simulink model "full_obs_res_gen_sim"  (R2020a)
settings: Solver=VariableStepAuto  StartTime=0.0  StopTime=15.0  RelTol=1e-3
values from neighbouring files (symbols this model uses):
  A = [ [0.5,1,0]; [1, 0, -1]; [1, 1, -0.5] ]    [init_demo_plant.m]    (also in init_demo_plant_2.m = [ [0.5,0.41,0.7]; [0.75, 0, -1.8]; [1.1, 0.8, -0.5] ])
  B = [ [1, -1]; [0, 1]; [1, 0] ]    [init_demo_plant.m]    (also in init_demo_plant_2.m = [ [0.1, -0.2, 0.3]; [0.5, 0.1, 0.35]; [1, 0, 0.7] ])
  C = [ [1, 0, 0]; [0, 0, 1] ]    [init_demo_plant.m]    (also in init_demo_plant_2.m = [ [1, 0, 0]; [0, 0, 1]; [0, 1, 0] ])
  D = [ [0, 0]; [0, 0] ]    [init_demo_plant.m]    (also in init_demo_plant_2.m = [ [0, 0, 0]; [0, 0, 0]; [0, 0, 0] ])
  E_d = [1; 0; 1]    [init_demo_plant.m]    (also in init_demo_plant_2.m = [ [0.1, 0.2, 0]; [0, 0.5, 0.2]; [1, 0.5, 0.7]])
  E_f = [0; 0; 1]    [init_demo_plant.m]    (also in init_demo_plant_2.m)
  F_d = [0; 0]    [init_demo_plant.m]    (also in init_demo_plant_2.m = [ [0, 0, 0]; [0, 0, 0]; [0, 0, 0] ])
  F_f = [1; 0]    [init_demo_plant.m]    (also in init_demo_plant_2.m = [0.2; 0.6; 0])
  L = place((A-E_d*M*C*A)', C', poles)'    [UIO_full_decoupling_res_gen.m]    (also in full_obs_res_gen.m = place(A', C', poles)')
  sigs = DemoSignals(m, mag_min, mag_max, n_d, n_f, stair_int, end_time)    [full_obs_res_gen.m]
  W = eye(q,p)    [UIO_full_decoupling_res_gen.m]    (also in full_obs_res_gen.m; parity_space_res_gen.m)
  x_0 = 5.*ones(3,1)    [UIO_full_decoupling_res_gen.m]    (also in full_obs_res_gen.m; parity_space_res_gen.m)
libraries: simulink x3
settings Model: Creator=faaizz  LastModifiedBy=faaizz

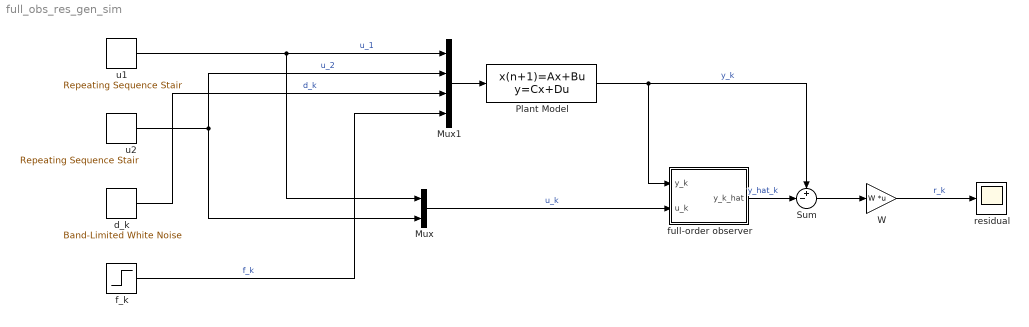
== system full_obs_res_gen_sim ==
  Mux : Mux  Inputs=2
  Mux1 : Mux
  Plant Model : DiscreteStateSpace  A=A  B=[ B, E_d, E_f ]  C=C  D=[D, F_d, F_f]  InitialCondition=x_0  SampleTime=-1
  Sum : Sum  Inputs=+-|
  W : Gain  Gain=W  Multiplication=Matrix(K*u)
  d_k : simulink/Sources/Band-Limited White Noise  Cov=sigs.disturbances.n_powers(1, :)  Ts=0.1  seed=sigs.disturbances.seeds(1,:)
  f_k : Step  Time=sigs.faults.times(1,:)  After=sigs.faults.amp  SampleTime=0
  full-order observer : Subsystem
  residual : Scope
  u1 : simulink/Sources/Repeating Sequence Stair  OutValues=sigs.inputs.signals(1, :)'  tsamp=sigs.inputs.k  OutMin=[]  OutMax=[]  OutDataTypeStr=double  OutputDataTypeScalingMode=double  OutDataType=fixdt(0,8)  ConRadixGroup=Best Precision: Vector-wise  OutScaling=2^-12
  u2 : simulink/Sources/Repeating Sequence Stair  OutValues=sigs.inputs.signals(2, :)'  tsamp=sigs.inputs.k  OutMin=[]  OutMax=[]  OutDataTypeStr=double  OutputDataTypeScalingMode=double  OutDataType=fixdt(0,8)  ConRadixGroup=Best Precision: Vector-wise  OutScaling=2^-12
  wires:
  u1/1 -> Mux/1, Mux1/1  "u_1"
  u2/1 -> Mux1/2, Mux/2  "u_2"
  Mux1/1 -> Plant Model/1
  d_k/1 -> Mux1/3  "d_k"
  f_k/1 -> Mux1/4  "f_k"
  Plant Model/1 -> full-order observer/1(y_k), Sum/1  "y_k"
  Mux/1 -> full-order observer/2(u_k)  "u_k"
  full-order observer/1(y_k_hat) -> Sum/2  "y_hat_k"
  Sum/1 -> W/1
  W/1 -> residual/1  "r_k"

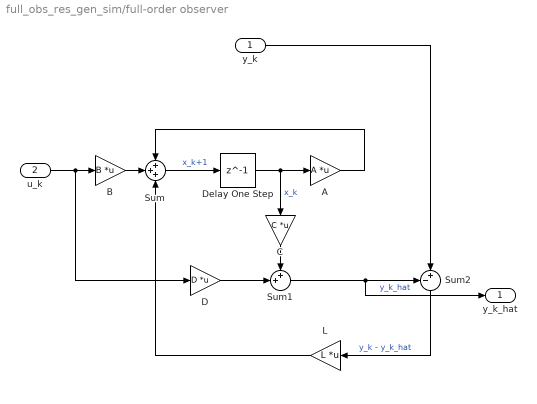
== system full_obs_res_gen_sim/full-order observer ==
  y_k : Inport
  u_k : Inport  Port=2
  A : Gain  Gain=A  Multiplication=Matrix(K*u)
  B : Gain  Gain=B  Multiplication=Matrix(K*u)
  C : Gain  Gain=C  Multiplication=Matrix(K*u)
  D : Gain  Gain=D  Multiplication=Matrix(K*u)
  Delay One Step : Delay  DelayLength=1
  L : Gain  Gain=L  Multiplication=Matrix(K*u)
  Sum : Sum  Inputs=+++
  Sum1 : Sum  Inputs=++|
  Sum2 : Sum  Inputs=-+|
  y_k_hat : Outport
  wires:
  y_k/1 -> Sum2/2
  Delay One Step/1 -> A/1, C/1  "x_k"
  Sum2/1 -> L/1  "y_k - y_k_hat"
  L/1 -> Sum/3
  A/1 -> Sum/1
  Sum1/1 -> y_k_hat/1, Sum2/1  "y_k_hat"
  Sum/1 -> Delay One Step/1  "x_k+1"
  B/1 -> Sum/2
  u_k/1 -> D/1, B/1
  C/1 -> Sum1/1
  D/1 -> Sum1/2
